simulink model "BT11_Dieukhienvitri_PID"  (R2022a)
settings: Solver=FixedStepAuto  StartTime=0.0  StopTime=20  FixedStep=0.01  RelTol=1e-3  EnableMultiTasking=on
libraries: arduinolib x3, arduinosensorlib x1
settings Model: ExtModeTrigDuration=2  Creator=quoc2  LastModifiedBy=kietn
settings OptimizationCC: EnhancedBackFolding=on  PassReuseOutputArgsAs=Individual arguments  ZeroExternalMemoryAtStartup=off  ZeroInternalMemoryAtStartup=off  MaxStackSize=64  OptimizeBlockOrder=speed  DifferentSizesBufferReuse=on  EfficientTunableParamExpr=on
settings DebuggingCC: ParameterTunabilityLossMsg=error
settings HardwareCC: ProdBitPerPointer=32  ProdBitPerSizeT=32  ProdBitPerPtrDiffT=32  ProdLargestAtomicInteger=Long  ProdLargestAtomicFloat=Double  ProdWordSize=32  ProdHWDeviceType=ARM Compatible->ARM Cortex
settings SFSimCC: MATLABDynamicMemAlloc=off
settings RTWCC: SystemTargetFile=ert.tlc  HardwareBoard=ESP32-WROOM(Arduino Compatible)  TLCOptions="-aInlineSetEventsForThisBaseRateFcn=TLC_FALSE -aSuppressMultiTaskScheduler=TLC_FALSE              -aRateBasedStepFcn=0"  TemplateMakefile=ert_default_tmf  Toolchain=ESP32  BuildConfiguration=Faster Runs
settings CodeAppCC: ForceParamTrailComments=on  IgnoreCustomStorageClasses=off  OperatorAnnotations=on  SimulinkDataObjDesc=on  SFDataObjDesc=on  InsertBlockDesc=on
settings ERTTargetCC: SupportContinuousTime=on  SupportVariableSizeSignals=on  ExtMode=on  ExtModeTransport=3  ExtModeStaticAlloc=on  ExtModeStaticAllocSize=65536  ExtModeMexFile=ext_xcp  ExtModeMexArgs=0 3 921600 'E:\Matlab2022a\PID.elf' 3 1000  ExtModeIntrfLevel=Level2 - Open

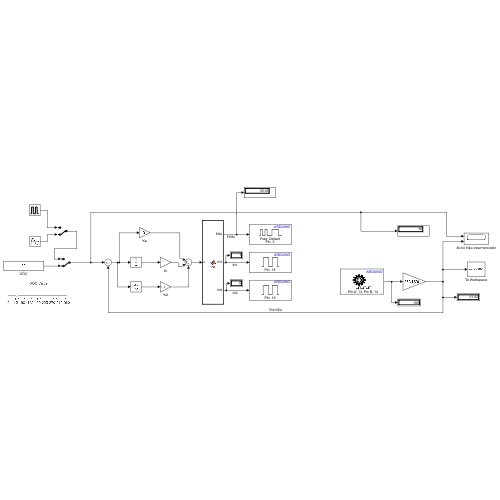
[thumbnail: Simulink's stored preview of the top-level diagram]
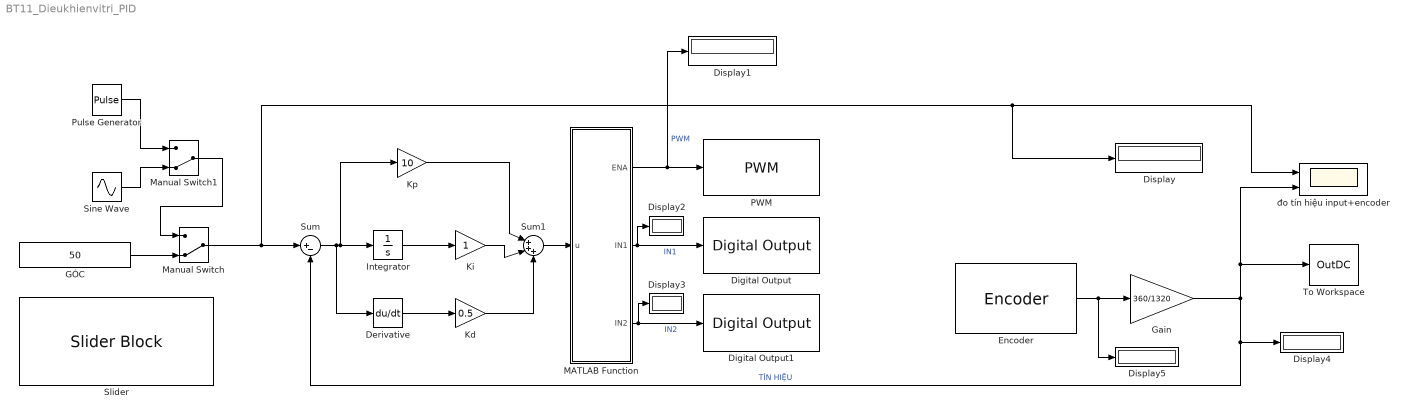
== system BT11_Dieukhienvitri_PID ==
  Derivative : Derivative
  Digital Output : arduinolib/Digital Output  pinNumber=18  Direction=output  blockPlatform=arduino
  Digital Output1 : arduinolib/Digital Output  pinNumber=19  Direction=output  blockPlatform=arduino
  Display{,1..5} (6 alike) : Display
  Encoder : arduinosensorlib/Encoder  InputA=13  InputB=14  Mode=No reset  SampleTime=-1
      settings: SourceProductBaseCode=ARDUINO
  Gain : Gain  Gain=360/1320
  GÓC : Constant  Value=50  VectorParams1D=off  OutDataTypeStr=uint16
  Integrator : Integrator
  Kd : Gain  Gain=0.5
  Ki : Gain
  Kp : Gain  Gain=10
  MATLAB Function : MATLAB Function  TreatAsAtomicUnit=on
  Manual Switch : ManualSwitch  CurrentSetting=0
  Manual Switch1 : ManualSwitch  CurrentSetting=0
  PWM : arduinolib/PWM  pinNumber=5  frequencyType=Default  desiredFrequency=490.2  achievableFrequency=490.2
  Pulse Generator : DiscretePulseGenerator  PulseType=Time based  Amplitude=300  Period=15  PulseWidth=50  PhaseDelay=-1
  Sine Wave : Sin  Amplitude=45  SampleTime=0
  Slider : SliderBlock  ScaleMax=360
  Sum : Sum  Inputs=|+-
  Sum1 : Sum  Inputs=|+++
  To Workspace : ToWorkspace  VariableName=OutDC  SampleTime=-1
      settings: Save2DSignal=2-D array (concatenate along first dimension)
  đo tín hiệu input+encoder : Scope  NumInputPorts=2
  wires:
  MATLAB Function/2(IN1) -> Display2/1, Digital Output/1  "IN1"
  MATLAB Function/3(IN2) -> Display3/1, Digital Output1/1  "IN2"
  Gain/1 -> Display4/1, Sum/2, To Workspace/1, đo tín hiệu input+encoder/2  "TÍN HIỆU"
  Encoder/1 -> Display5/1, Gain/1
  GÓC/1 -> Manual Switch/2
  Manual Switch/1 -> Display/1, đo tín hiệu input+encoder/1, Sum/1
  Pulse Generator/1 -> Manual Switch1/1
  Sine Wave/1 -> Manual Switch1/2
  Manual Switch1/1 -> Manual Switch/1
  MATLAB Function/1(ENA) -> Display1/1, PWM/1  "PWM"
  Sum/1 -> Derivative/1, Integrator/1, Kp/1
  Sum1/1 -> MATLAB Function/1(u)
  Kp/1 -> Sum1/1
  Derivative/1 -> Kd/1
  Integrator/1 -> Ki/1
  Kd/1 -> Sum1/3
  Ki/1 -> Sum1/2

== matlab function BT11_Dieukhienvitri_PID/MATLAB Function ==
  data: u input; ENA output; IN1 output; IN2 output
function [ENA,IN1,IN2] = fcn(u)

ENA=abs(u);
if u<0 
    IN1=1; IN2=0;
elseif u>0
    IN1=0; IN2=1;
else 
    IN1=0; IN2=0;
end
